simulink model "blocks"  (R2019a)
settings: Solver=VariableStepAuto  StartTime=0.0  StopTime=10.0  RelTol=1e-3
settings Model: Creator=adeye  LastModifiedBy=adeye

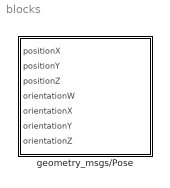
== system blocks ==
  geometry_msgs/Pose : Subsystem  mask{topic='/gnss_pose_simulink', message_type='geometry_msgs/Pose', port=9090, timeout=2}
      mask prompts: topic "Topic name"; message_type "Message type"; timeout "Timeout (s)"

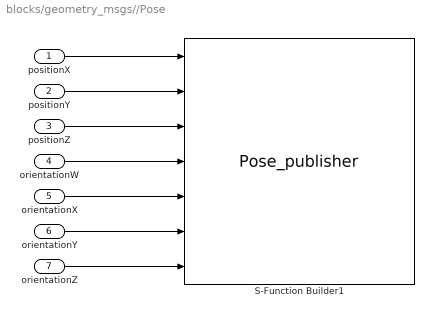
== system blocks/geometry_msgs//Pose ==
  positionX : Inport
  positionY : Inport  Port=2
  positionZ : Inport  Port=3
  orientationW : Inport  Port=4
  orientationX : Inport  Port=5
  orientationY : Inport  Port=6
  orientationZ : Inport  Port=7
  S-Function Builder1 : S-Function  InitFcn=try, set_param(gcb,'FunctionName','Pose_publisher'), end  FunctionName=Pose_publisher  Parameters=int8(topic),int8(message_type),port,timeout  SFunctionModules=Pose_publisher_wrapper rosbridge_functions  SFunctionDeploymentMode=off  EnableBusSupport=off  mask(S-Function Builder){}
      mask help: Simulink:masks:SFunctionBuilder_MD
      mask init:
      | val = [[.9  0.75 0.75 1 1 .9 .9 1]',[1 1 0.75 0.75 .9 .9 1 .9]'];try , sys = get_param(gcb,'SfunBuilderFcnName');if isempty(sys), sys = get_param(gcb,'FunctionName'); end,catch, sys = get_param(gcb,'FunctionName'); end
      settings: CopyFcn=set_param(gcbh,'LinkStatus','none')  PreSaveFcn=try, set_param(gcb,'FunctionName','Pose_publisher'), end  OpenFcn=sfunctionwizard(gcbh)
      mask Display: plot(val(:,1),val(:,2)),disp(sys), port_label('input',1,'positionX'), port_label('input',2,'positionY'), port_label('input',3,'positionZ'), port_label('input',4,'orientationW'), port_label('input',5,'orientationX'), port_label('input',6,'orientationY'), port_label('input',7,'orientationZ')
  wires:
  positionX/1 -> S-Function Builder1/1
  positionY/1 -> S-Function Builder1/2
  positionZ/1 -> S-Function Builder1/3
  orientationW/1 -> S-Function Builder1/4
  orientationX/1 -> S-Function Builder1/5
  orientationY/1 -> S-Function Builder1/6
  orientationZ/1 -> S-Function Builder1/7
